simulink model "carga_suspendida"  (R2019a)
settings: Solver=VariableStepAuto  StartTime=0.0  StopTime=10.0  RelTol=1e-3
values from neighbouring files (symbols this model uses):
  b_cx = 1.0e6    (= 1000000)    [parametros.m]
  b_cy = 1.0e7    (= 10000000)    [parametros.m]
  g = 9.80665    [parametros.m]
  K_cy = 1.8e9    (= 1800000000)    [parametros.m]
  x_l0 = x_t0    (= -30)    [parametros.m]
  y_l0 = y_h0    (= 2.5)    [parametros.m]
  Y_t0 = 45.0    (= 45)    [parametros.m]
settings Model: Creator=Facundo  LastModifiedBy=Facundo

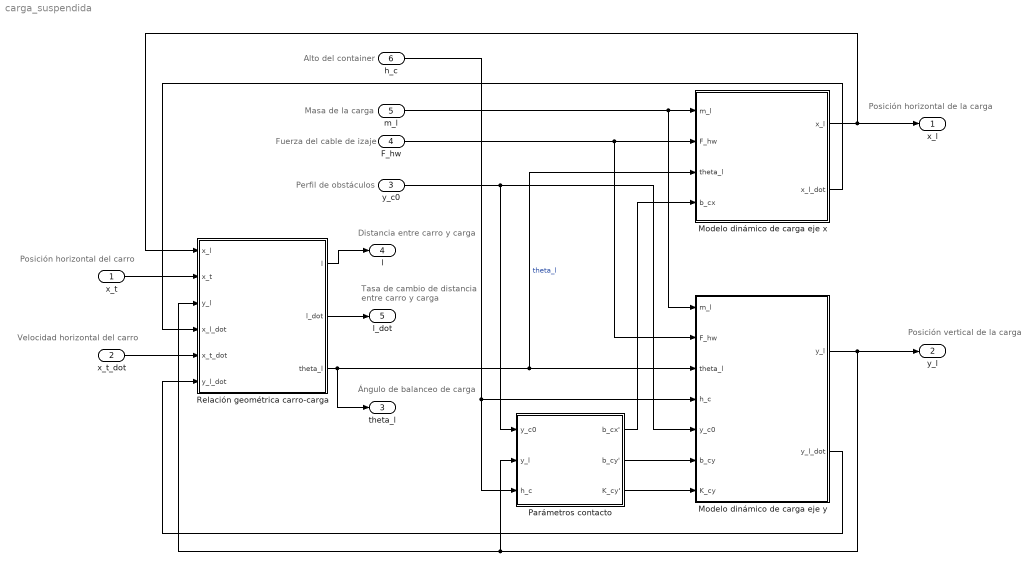
== system carga_suspendida ==
  note: Alto del container
  note: Ángulo de balanceo de carga
  note: Perfil de obstáculos
  note: Tasa de cambio de distancia
      | entre carro y carga
  note: Posición vertical de la carga
  note: Posición horizontal del carro
  note: Velocidad horizontal del carro
  note: Fuerza del cable de izaje
  note: Distancia entre carro y carga
  note: Posición horizontal de la carga
  note: Masa de la carga
  x_t : Inport  OutDataTypeStr=double  PortDimensions=1  SampleTime=0
  x_t_dot : Inport  Port=2  OutDataTypeStr=double  PortDimensions=1  SampleTime=0
  y_c0 : Inport  Port=3  OutDataTypeStr=double  PortDimensions=1  SampleTime=0
  F_hw : Inport  Port=4  OutDataTypeStr=double  PortDimensions=1  SampleTime=0
  m_l : Inport  Port=5  OutDataTypeStr=double  PortDimensions=1  SampleTime=0
  h_c : Inport  Port=6  OutDataTypeStr=double  PortDimensions=1  SampleTime=0
  Modelo dinámico de carga eje x : Subsystem
  Modelo dinámico de carga eje y : Subsystem
  Parámetros contacto : Subsystem
  Relación geométrica carro-carga : Subsystem
  x_l : Outport  OutDataTypeStr=double  PortDimensions=1  SampleTime=0
  y_l : Outport  Port=2  OutDataTypeStr=double  PortDimensions=1  SampleTime=0
  theta_l : Outport  Port=3  OutDataTypeStr=double  PortDimensions=1  SampleTime=0
  l : Outport  Port=4  OutDataTypeStr=double  PortDimensions=1  SampleTime=0
  l_dot : Outport  Port=5  OutDataTypeStr=double  PortDimensions=1  SampleTime=0
  wires:
  x_t/1 -> Relación geométrica carro-carga/2(x_t)
  Relación geométrica carro-carga/3(theta_l) -> theta_l/1, Modelo dinámico de carga eje x/3(theta_l), Modelo dinámico de carga eje y/3(theta_l)  "theta_l"
  Modelo dinámico de carga eje y/2(y_l_dot) -> Relación geométrica carro-carga/6(y_l_dot)
  Modelo dinámico de carga eje x/1(x_l) -> x_l/1, Relación geométrica carro-carga/1(x_l)
  Parámetros contacto/3(K_cy') -> Modelo dinámico de carga eje y/7(K_cy)
  Parámetros contacto/1(b_cx') -> Modelo dinámico de carga eje x/4(b_cx)
  Relación geométrica carro-carga/2(l_dot) -> l_dot/1
  Modelo dinámico de carga eje y/1(y_l) -> y_l/1, Relación geométrica carro-carga/3(y_l), Parámetros contacto/2(y_l)
  m_l/1 -> Modelo dinámico de carga eje y/1(m_l), Modelo dinámico de carga eje x/1(m_l)
  Relación geométrica carro-carga/1(l) -> l/1
  F_hw/1 -> Modelo dinámico de carga eje y/2(F_hw), Modelo dinámico de carga eje x/2(F_hw)
  h_c/1 -> Modelo dinámico de carga eje y/4(h_c), Parámetros contacto/3(h_c)
  Modelo dinámico de carga eje x/2(x_l_dot) -> Relación geométrica carro-carga/4(x_l_dot)
  Parámetros contacto/2(b_cy') -> Modelo dinámico de carga eje y/6(b_cy)
  x_t_dot/1 -> Relación geométrica carro-carga/5(x_t_dot)
  y_c0/1 -> Parámetros contacto/1(y_c0), Modelo dinámico de carga eje y/5(y_c0)

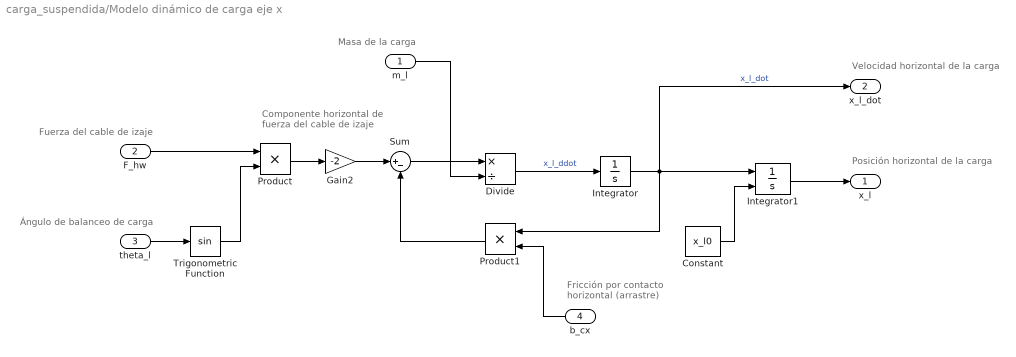
== system carga_suspendida/Modelo dinámico de carga eje x ==
  note: Componente horizontal de
      | fuerza del cable de izaje
  note: Posición horizontal de la carga
  note: Velocidad horizontal de la carga
  note: Fuerza del cable de izaje
  note: Masa de la carga
  note: Fricción por contacto
      | horizontal (arrastre)
  note: Ángulo de balanceo de carga
  m_l : Inport  OutDataTypeStr=double  PortDimensions=1  SampleTime=0
  F_hw : Inport  Port=2  OutDataTypeStr=double  PortDimensions=1  SampleTime=0
  theta_l : Inport  Port=3  OutDataTypeStr=double  PortDimensions=1  SampleTime=0
  b_cx : Inport  Port=4  OutDataTypeStr=double  PortDimensions=1  SampleTime=0
  Constant : Constant  Value=x_l0
  Divide : Product  Inputs=*/
  Gain2 : Gain  Gain=-2
  Integrator : Integrator
  Integrator1 : Integrator  InitialConditionSource=external
  Product : Product
  Product1 : Product
  Sum : Sum  Inputs=|+-
  Trigonometric Function : Trigonometry
  x_l : Outport  OutDataTypeStr=double  PortDimensions=1  SampleTime=0
  x_l_dot : Outport  Port=2  OutDataTypeStr=double  PortDimensions=1  SampleTime=0
  wires:
  F_hw/1 -> Product/1
  Product1/1 -> Sum/2
  theta_l/1 -> Trigonometric Function/1
  b_cx/1 -> Product1/2
  Sum/1 -> Divide/1
  Integrator/1 -> x_l_dot/1, Integrator1/1, Product1/1  "x_l_dot"
  Product/1 -> Gain2/1
  Divide/1 -> Integrator/1  "x_l_ddot"
  Constant/1 -> Integrator1/2
  Integrator1/1 -> x_l/1
  Gain2/1 -> Sum/1
  m_l/1 -> Divide/2
  Trigonometric Function/1 -> Product/2

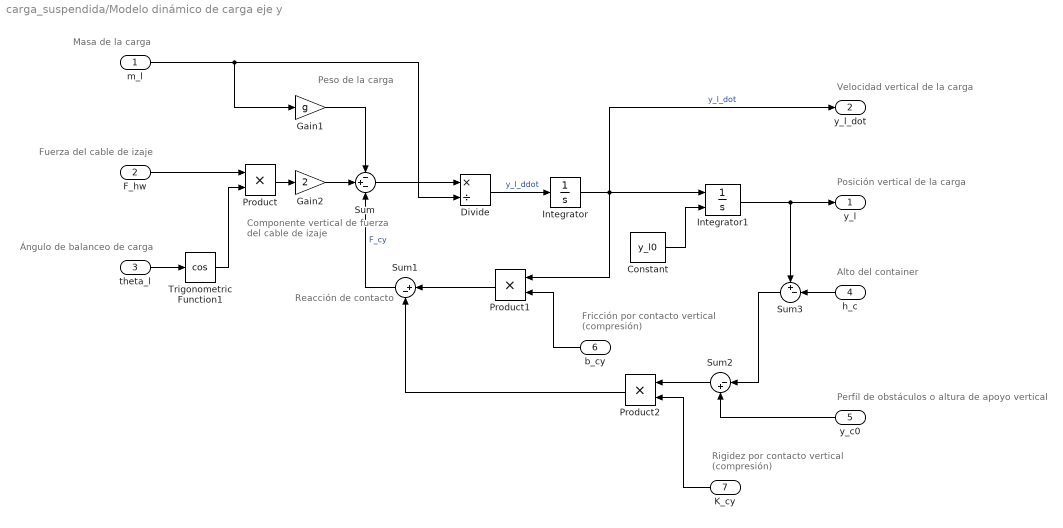
== system carga_suspendida/Modelo dinámico de carga eje y ==
  note: Reacción de contacto
  note: Peso de la carga
  note: Componente vertical de
      | fuerza del cable de izaje
  note: Posición vertical de la carga
  note: Velocidad vertical de la carga
  note: Fricción por contacto
      | vertical (compresión)
  note: Rigidez por contacto
      | vertical (compresión)
  note: Masa de la carga
  note: Fuerza del cable de izaje
  note: Perfil de obstáculos o altura de apoyo vertical
  note: Alto del container
  note: Ángulo de balanceo de carga
  m_l : Inport  OutDataTypeStr=double  PortDimensions=1  SampleTime=0
  F_hw : Inport  Port=2  OutDataTypeStr=double  PortDimensions=1  SampleTime=0
  theta_l : Inport  Port=3  OutDataTypeStr=double  PortDimensions=1  SampleTime=0
  h_c : Inport  Port=4  OutDataTypeStr=double  PortDimensions=1  SampleTime=0
  y_c0 : Inport  Port=5  OutDataTypeStr=double  PortDimensions=1  SampleTime=0
  b_cy : Inport  Port=6  OutDataTypeStr=double  PortDimensions=1  SampleTime=0
  K_cy : Inport  Port=7  OutDataTypeStr=double  PortDimensions=1  SampleTime=0
  Constant : Constant  Value=y_l0
  Divide : Product  Inputs=*/
  Gain1 : Gain  Gain=g
  Gain2 : Gain  Gain=2
  Integrator : Integrator
  Integrator1 : Integrator  InitialConditionSource=external
  Product : Product
  Product1 : Product
  Product2 : Product
  Sum : Sum  Inputs=-+-
  Sum1 : Sum  Inputs=|+-
  Sum2 : Sum  Inputs=|-+
  Sum3 : Sum  Inputs=+-|
  Trigonometric Function1 : Trigonometry  Operator=cos
  y_l : Outport  OutDataTypeStr=double  PortDimensions=1  SampleTime=0
  y_l_dot : Outport  Port=2  OutDataTypeStr=double  PortDimensions=1  SampleTime=0
  wires:
  F_hw/1 -> Product/1
  theta_l/1 -> Trigonometric Function1/1
  b_cy/1 -> Product1/2
  Integrator/1 -> y_l_dot/1, Integrator1/1, Product1/1  "y_l_dot"
  Divide/1 -> Integrator/1  "y_l_ddot"
  Constant/1 -> Integrator1/2
  Integrator1/1 -> y_l/1, Sum3/1
  Product/1 -> Gain2/1
  Product1/1 -> Sum1/1
  Sum1/1 -> Sum/3  "F_cy"
  Gain1/1 -> Sum/1
  y_c0/1 -> Sum2/2
  Sum2/1 -> Product2/1
  K_cy/1 -> Product2/2
  Product2/1 -> Sum1/2
  Gain2/1 -> Sum/2
  Sum/1 -> Divide/1
  m_l/1 -> Gain1/1, Divide/2
  h_c/1 -> Sum3/2
  Sum3/1 -> Sum2/1
  Trigonometric Function1/1 -> Product/2

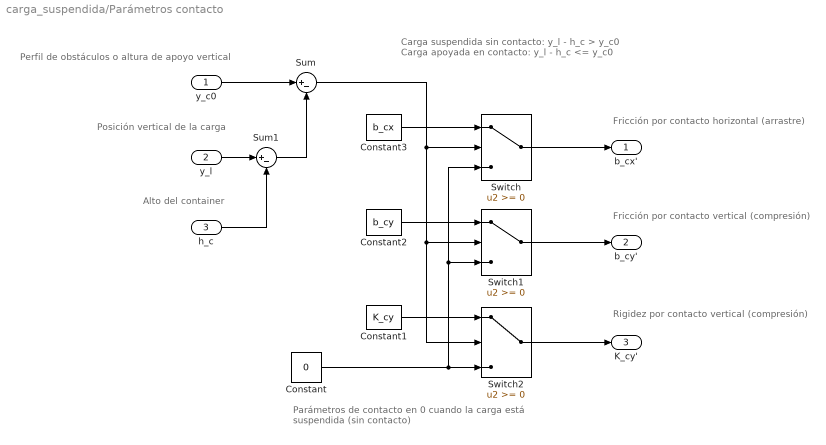
== system carga_suspendida/Parámetros contacto ==
  note: Fricción por contacto horizontal (arrastre)
  note: Fricción por contacto vertical (compresión)
  note: Rigidez por contacto vertical (compresión)
  note: Perfil de obstáculos o altura de apoyo vertical
  note: Posición vertical de la carga
  note: Alto del container
  note: Parámetros de contacto en 0
      | cuando la carga está suspendida (sin contacto)
  note: Carga suspendida sin contacto: y_l - h_c > y_c0
      | Carga apoyada en contacto: y_l - h_c <= y_c0
  y_c0 : Inport  OutDataTypeStr=double  PortDimensions=1  SampleTime=0
  y_l : Inport  Port=2  OutDataTypeStr=double  PortDimensions=1  SampleTime=0
  h_c : Inport  Port=3  OutDataTypeStr=double  PortDimensions=1  SampleTime=0
  Constant : Constant  Value=0
  Constant1 : Constant  Value=K_cy
  Constant2 : Constant  Value=b_cy
  Constant3 : Constant  Value=b_cx
  Sum : Sum  Inputs=|+-
  Sum1 : Sum  Inputs=|+-
  Switch : Switch
  Switch1 : Switch
  Switch2 : Switch
  b_cx' : Outport  OutDataTypeStr=double  PortDimensions=1  SampleTime=0
  b_cy' : Outport  Port=2  OutDataTypeStr=double  PortDimensions=1  SampleTime=0
  K_cy' : Outport  Port=3  OutDataTypeStr=double  PortDimensions=1  SampleTime=0
  wires:
  y_c0/1 -> Sum/1
  Constant2/1 -> Switch1/1
  Constant1/1 -> Switch2/1
  Switch/1 -> b_cx'/1
  Sum/1 -> Switch1/2, Switch2/2, Switch/2
  Switch2/1 -> K_cy'/1
  Switch1/1 -> b_cy'/1
  Constant/1 -> Switch/3, Switch1/3, Switch2/3
  Constant3/1 -> Switch/1
  Sum1/1 -> Sum/2
  y_l/1 -> Sum1/1
  h_c/1 -> Sum1/2

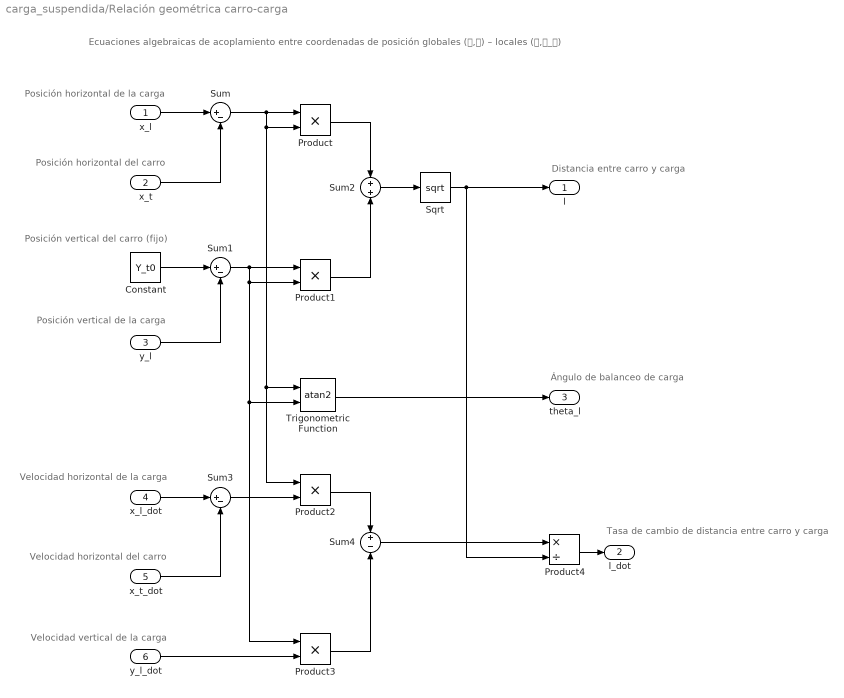
== system carga_suspendida/Relación geométrica carro-carga ==
  note: Ecuaciones algebraicas de acoplamiento entre coordenadas de posición globales (𝑥,𝑦) – locales (𝑙,𝜃_𝑙)
  note: Posición horizontal de la carga
  note: Posición horizontal del carro
  note: Posición vertical del carro (fijo)
  note: Posición vertical de la carga
  note: Distancia entre carro y carga
  note: Tasa de cambio de distancia entre carro y carga
  note: Ángulo de balanceo de carga
  note: Velocidad horizontal de la carga
  note: Velocidad horizontal del carro
  note: Velocidad vertical de la carga
  x_l : Inport
  x_t : Inport  Port=2
  y_l : Inport  Port=3
  x_l_dot : Inport  Port=4
  x_t_dot : Inport  Port=5
  y_l_dot : Inport  Port=6
  Constant : Constant  Value=Y_t0
  Product{,1..3} (4 alike) : Product
  Product4 : Product  Inputs=*/
  Sqrt : Sqrt  SaturateOnIntegerOverflow=on
  Sum : Sum  Inputs=|+-
  Sum1 : Sum  Inputs=|+-
  Sum2 : Sum  Inputs=+|+
  Sum3 : Sum  Inputs=|+-
  Sum4 : Sum  Inputs=+|-
  Trigonometric Function : Trigonometry  Operator=atan2
  l : Outport
  l_dot : Outport  Port=2
  theta_l : Outport  Port=3
  wires:
  x_t/1 -> Sum/2
  x_l/1 -> Sum/1
  Sum/1 -> Product/1, Product2/1, Trigonometric Function/1, Product/2
  Product/1 -> Sum2/1
  y_l/1 -> Sum1/2
  Sum1/1 -> Product1/1, Product3/1, Trigonometric Function/2, Product1/2
  Constant/1 -> Sum1/1
  Product1/1 -> Sum2/2
  Sum2/1 -> Sqrt/1
  Trigonometric Function/1 -> theta_l/1
  x_l_dot/1 -> Sum3/1
  x_t_dot/1 -> Sum3/2
  Sum3/1 -> Product2/2
  y_l_dot/1 -> Product3/2
  Product2/1 -> Sum4/1
  Product3/1 -> Sum4/2
  Sum4/1 -> Product4/1
  Product4/1 -> l_dot/1
  Sqrt/1 -> Product4/2, l/1
